simulink library "hdlssclib"  (R2019a)
settings: Solver=VariableStepAuto  StartTime=0.0  StopTime=10.0  RelTol=1e-3
undefined symbols (not defined in the file or in its folder): constMatrix
libraries: $bdroot x4
settings Model: Creator=The MathWorks, Inc.  LastModifiedBy=The MathWorks, Inc.
settings DataIOCC: ReturnWorkspaceOutputs=off
settings DebuggingCC: ArithmeticOperatorsInVariantConditions=warning
settings SFSimCC: SimUseLocalCustomCode=off
settings RTWCC: RTWUseLocalCustomCode=off
settings CodeAppCC: StateflowObjectComments=on
settings GRTTargetCC: TargetLangStandard=C89/C90 (ANSI)
settings ConfigComp: CovMetricSettings=dsw  CovHtmlReporting=on  CovSaveCumulativeToWorkspaceVar=on  CovSaveSingleToWorkspaceVar=on  CovShowResultsExplorer=off  CovExternalEMLEnable=off

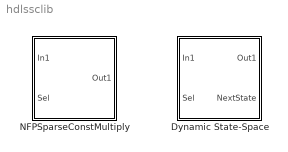
== system hdlssclib ==
  Dynamic State-Space : Subsystem  mask{A=1, B=1, C=1, D=1, X0=0}
      mask prompts: X0 "Initial conditions:"
      mask init:
      | % Dynamic State-Space block configuration
      | % the Dynamic State-Space block has multiple possible configurations based
      | % on the mask parameter values
      | % the Dynamic State-Space block implements the following equations:
      | % NextState     = A * State + B * In1 -> state update equation
      | % Out1          = C * State + D * In1 -> output equation
      | % State <- NextState
      | %
      | % where A, B, C, and D are mask parameters
      | % State represents the current internal state
      | % NextState and Out1 are block outputs
      | % In1 and Sel are block inputs
      | % Sel indexes into dimension 3 of the mask parameters A, B, C, and D
      | 
      | % determine the block configuration from the mask parameter values
      | % three configurations of the Dynamic State-Space block are currently
      | % implemented
      | % configuration 1 - nonzero A,B,C,D
      | % configuration 2 - nonzero A,B,C and zero D
      | % configuration 3 - nonzero D and zero A,B,C
      | 
      | % determine nonzero mask parameters
      | isNonZeroA = any(A(:));
      | isNonZeroB = any(B(:));
      | isNonZeroC = any(C(:));
      | isNonZeroD = any(D(:));
      | 
      | if all([isNonZeroA isNonZeroB isNonZeroC isNonZeroD])
      |     % configuration 1
      |     % x(n+1)    = A*x(n) + B*u(n)
      |     % y(n)      = C*x(n) + D*u(n)
      |     config = 1;
      | elseif all([isNonZeroA isNonZeroB isNonZeroC ~isNonZeroD])
      |     % configuration 2
      |     % x(n+1)    = A*x(n) + B*u(n)
      |     % y(n)      = C*x(n)
      |     config = 2;
      | elseif all([~isNonZeroA ~isNonZeroB ~isNonZeroC isNonZeroD])
      |     % configuration 3
      |     % x(n+1)    = 0
      |     % y(n)      = D*u(n)
      |     config = 3;
      | else
      |     % unimplemented configuration
      |     % default implementation = configuration 1
      |     config = 1;
      | end
      | 
      | % top level block - Dynamic State-Space
      | topBlk = gcb;
      | 
      | % Dynamic State-Space block inports and outports
      | topInports = find_system(topBlk,'LookUnderMasks','all','FollowLinks','on','SearchDepth','1','BlockType','Inport');
      | topOutports = find_system(topBlk,'LookUnderMasks','all','FollowLinks','on','SearchDepth','1','BlockType','Outport');
      | 
      | % blocks inside the Dynamic State-Space block
      | % (not all blocks are present in every configuration)
      | % Name: block name, Position: block position
      | blks = [];
      | % NFPSparseConstMultiply blocks to implement floating point multiplications
      | blks(1).Name = 'NFPMulA';
      | blks(1).Position = [110 170 190 250];
      | blks(2).Name = 'NFPMulB';
      | blks(2).Position = [110 30 190 110];
      | blks(3).Name = 'NFPMulC';
      | blks(3).Position = [410 85 490 165];
      | blks(4).Name = 'NFPMulD';
      | blks(4).Position = [410 -40 490 40];
      | % Sum blocks to implement floating point additions
      | blks(5).Name = 'SumAB';
      | blks(5).Position = [230 55 260 85];
      | blks(6).Name = 'SumCD';
      | blks(6).Position = [520 -15 550 15];
      | % Unit delay block to implement the state
      | blks(7).Name = 'State';
      | blks(7).Position = [295 53 330 87];
      | 
      | % delete all blocks before redrawing
      | nfpMulBlks = find_system(topBlk,'LookUnderMasks','all','FollowLinks','on','SearchDepth','1','ReferenceBlock','hdlssclib/NFPSparseConstMultiply');
      | sumBlks = find_system(topBlk,'LookUnderMasks','all','FollowLinks','on','SearchDepth','1','BlockType','Sum');
      | delayBlks = find_system(topBlk,'LookUnderMasks','all','FollowLinks','on','SearchDepth','1','BlockType','UnitDelay');
      | constBlks = find_system(topBlk,'LookUnderMasks','all','FollowLinks','on','SearchDepth','1','BlockType','Constant');
      | trmtBlks = find_system(topBlk,'LookUnderMasks','all','FollowLinks','on','SearchDepth','1','BlockType','Terminator');
      | deleteBlks = [nfpMulBlks; sumBlks; delayBlks; constBlks; trmtBlks];
      | for ii = 1:numel(deleteBlks)
      |     hLines = get_param(deleteBlks{ii},'LineHandles');
      |     % get connected inport lines. this handles the situation when a block
      |     % inport is unconnected.
      |     inports = hLines.Inport(hLines.Inport ~= -1);
      |     % get connected outport lines. this handles the situation when a block
      |     % outport is unconnected.
      |     outports = hLines.Outport(hLines.Outport ~= -1);
      |     % delete inport connections
      |     delete_line(inports);
      |     % delete outport connections
      |     delete_line(outports);
      |     % delete the block
      |     delete_block(deleteBlks{ii});
      | end
      | 
      | if config == 1
      |     % configuration 1
      |     % x(n+1)    = A*x(n) + B*u(n)
      |     % y(n)      = C*x(n) + D*u(n)
      |     
      |     % add NFPMulA block to perform A*x(n)
      |     add_block('hdlssclib/NFPSparseConstMultiply',[topBlk '/' blks(1).Name],'Position',blks(1).Position);
      |     set_param([topBlk '/' blks(1).Name],'constMatrix','A');
      |     % add NFPMulB block to perform B*u(n)
      |     add_block('hdlssclib/NFPSparseConstMultiply',[topBlk '/' blks(2).Name],'Position',blks(2).Position);
      |     set_param([topBlk '/' blks(2).Name],'constMatrix','B');
      |     % add sum block to perform A*x(n) + B*u(n)
      |     add_block('simulink/Math Operations/Sum',[topBlk '/' blks(5).Name],'Position',blks(5).Position,'InputSameDT','on');
      |     % add unit delay block to store the state
      |     add_block('simulink/Discrete/Unit Delay',[topBlk '/' blks(7).Name],'Position',blks(7).Position);
      |     set_param([topBlk '/' blks(7).Name],'InitialCondition','X0');
      |     % connect NFPMulA and NFPMulB outputs to SumAB inputs
      |     add_line(topBlk,[blks(1).Name '/1'],[blks(5).Name '/2'],'autorouting','on');
      |     add_line(topBlk,[blks(2).Name '/1'],[blks(5).Name '/1'],'autorouting','on');
      |     % connect sumAB output to State input
      |     add_line(topBlk,[blks(5).Name '/1'],[blks(7).Name '/1'],'autorouting','on');
      |     % connect State output to NFPMulA input 'In1'
      |     add_line(topBlk,[blks(7).Name '/1'],[blks(1).Name '/1'],'autorouting','on');
      |     % connect Dynamic State-Space input 'In1' to NFPMulB input 'In1'
      |     add_line(topBlk,[get_param(topInports{1},'Name') '/1'],[blks(2).Name '/1'],'autorouting','on');
      |     % connect Dynamic State-Space input 'Sel' to NFPMulA and NFPMulB inputs
      |     % 'Sel'
      |     add_line(topBlk,[get_param(topInports{2},'Name') '/1'],[blks(1).Name '/2'],'autorouting','on');
      |     add_line(topBlk,[get_param(topInports{2},'Name') '/1'],[blks(2).Name '/2'],'autorouting','on');
      |     % add NFPMulC block to perform C*x(n)
      |     add_block('hdlssclib/NFPSparseConstMultiply',[topBlk '/' blks(3).Name],'Position',blks(3).Position);
      |     set_param([topBlk '/' blks(3).Name],'constMatrix','C');
      |     % add NFPMulD block to perform D*u(n)
      |     add_block('hdlssclib/NFPSparseConstMultiply',[topBlk '/' blks(4).Name],'Position',blks(4).Position);
      |     set_param([topBlk '/' blks(4).Name],'constMatrix','D');
      |     % add sum block to perform C*x(n) + D*u(n)
      |     add_block('simulink/Math Operations/Sum',[topBlk '/' blks(6).Name],'Position',blks(6).Position,'InputSameDT','on');
      |     % connect NFPMulC and NFPMulD outputs to SumCD inputs
      |     add_line(topBlk,[blks(3).Name '/1'],[blks(6).Name '/2'],'autorouting','on');
      |     add_line(topBlk,[blks(4).Name '/1'],[blks(6).Name '/1'],'autorouting','on');
      |     % connect State output to NFPMulC input 'In1'
      |     add_line(topBlk,[blks(7).Name '/1'],[blks(3).Name '/1'],'autorouting','on');
      |     % connect Dynamic State-Space input 'In1' to NFPMulD input 'In1'
      |     add_line(topBlk,[get_param(topInports{1},'Name') '/1'],[blks(4).Name '/1'],'autorouting','on');
      |     % connect Dynamic State-Space input 'Sel' to NFPMulC and NFPMulD inputs
      |     % 'Sel'
      |     add_line(topBlk,[get_param(topInports{2},'Name') '/1'],[blks(3).Name '/2'],'autorouting','on');
      |     add_line(topBlk,[get_param(topInports{2},'Name') '/1'],[blks(4).Name '/2'],'autorouting','on');
      |     % connect State output to Dynamic State-Space output 'NextState'
      |     add_line(topBlk,[blks(7).Name '/1'],[get_param(topOutports{2},'Name') '/1'],'autorouting','on');
      |     % connect SumCD output to Dynamic State-Space output 'Out1'
      |     add_line(topBlk,[blks(6).Name '/1'],[get_param(topOutports{1},'Name') '/1'],'autorouting','on');
      |     
      | elseif config == 2
      |     % configuration 2
      |     % x(n+1)    = A*x(n) + B*u(n)
      |     % y(n)      = C*x(n)
      |     
      |     % add NFPMulA block to perform A*x(n)
      |     add_block('hdlssclib/NFPSparseConstMultiply',[topBlk '/' blks(1).Name],'Position',blks(1).Position);
      |     set_param([topBlk '/' blks(1).Name],'constMatrix','A');
      |     % add NFPMulB block to perform B*u(n)
      |     add_block('hdlssclib/NFPSparseConstMultiply',[topBlk '/' blks(2).Name],'Position',blks(2).Position);
      |     set_param([topBlk '/' blks(2).Name],'constMatrix','B');
      |     % add sum block to perform A*x(n) + B*u(n)
      |     add_block('simulink/Math Operations/Sum',[topBlk '/' blks(5).Name],'Position',blks(5).Position,'InputSameDT','on');
      |     % add unit delay block to store the state
      |     add_block('simulink/Discrete/Unit Delay',[topBlk '/' blks(7).Name],'Position',blks(7).Position);
      |     set_param([topBlk '/' blks(7).Name],'InitialCondition','X0');
      |     % connect NFPMulA and NFPMulB outputs to SumAB inputs
      |     add_line(topBlk,[blks(1).Name '/1'],[blks(5).Name '/2'],'autorouting','on');
      |     add_line(topBlk,[blks(2).Name '/1'],[blks(5).Name '/1'],'autorouting','on');
      |     % connect sumAB output to State input
      |     add_line(topBlk,[blks(5).Name '/1'],[blks(7).Name '/1'],'autorouting','on');
      |     % connect State output to NFPMulA input 'In1'
      |     add_line(topBlk,[blks(7).Name '/1'],[blks(1).Name '/1'],'autorouting','on');
      |     % connect Dynamic State-Space input 'In1' to NFPMulB input 'In1'
      |     add_line(topBlk,[get_param(topInports{1},'Name') '/1'],[blks(2).Name '/1'],'autorouting','on');
      |     % connect Dynamic State-Space input 'Sel' to NFPMulA and NFPMulB inputs
      |     % 'Sel'
      |     add_line(topBlk,[get_param(topInports{2},'Name') '/1'],[blks(1).Name '/2'],'autorouting','on');
      |     add_line(topBlk,[get_param(topInports{2},'Name') '/1'],[blks(2).Name '/2'],'autorouting','on');
      |     % add NFPMulC block to perform C*x(n)
      |     add_block('hdlssclib/NFPSparseConstMultiply',[topBlk '/' blks(3).Name],'Position',blks(3).Position);
      |     set_param([topBlk '/' blks(3).Name],'constMatrix','C');
      |     % connect State output to NFPMulC input 'In1'
      |     add_line(topBlk,[blks(7).Name '/1'],[blks(3).Name '/1'],'autorouting','on');
      |     % connect Dynamic State-Space input 'Sel' to NFPMulC input 'Sel'
      |     add_line(topBlk,[get_param(topInports{2},'Name') '/1'],[blks(3).Name '/2'],'autorouting','on');
      |     % connect State output to Dynamic State-Space output 'NextState'
      |     add_line(topBlk,[blks(7).Name '/1'],[get_param(topOutports{2},'Name') '/1'],'autorouting','on');
      |     % connect NFPMulC output to Dynamic State-Space output 'Out1'
      |     add_line(topBlk,[blks(3).Name '/1'],[get_param(topOutports{1},'Name') '/1'],'autorouting','on');
      |     
      | else
      |     % configuration 3
      |     % x(n+1)    = 0
      |     % y(n)      = D*u(n)
      |     
      |     % add NFPMulD block to perform D*u(n)
      |     add_block('hdlssclib/NFPSparseConstMultiply',[topBlk '/' blks(4).Name],'Position',blks(4).Position);
      |     set_param([topBlk '/' blks(4).Name],'constMatrix','D');
      |     % connect Dynamic State-Space input 'In1' to NFPMulD input 'In1'
      |     add_line(topBlk,[get_param(topInports{1},'Name') '/1'],[blks(4).Name '/1'],'autorouting','on');
      |     % connect Dynamic State-Space input 'Sel' to NFPMulD input 'Sel'
      |     add_line(topBlk,[get_param(topInports{2},'Name') '/1'],[blks(4).Name '/2'],'autorouting','on');
      |     % connect NFPMulD output to Dynamic State-Space output 'Out1'
      |     add_line(topBlk,[blks(4).Name '/1'],[get_param(topOutports{1},'Name') '/1'],'autorouting','on');
      |     % connect Dynamic State-Space output 'NextState' to a constant block
      |     % with 0 value
      |     add_block('simulink/Sources/Constant',[topBlk '/Constant1'],...
      |         'Position',[525 -85 545 -65],...
      |         'Value', '0',...
      |         'SampleTime','-1',...
      |         'OutDataTypeStr','single');
      |     add_line(topBlk,'Constant1/1',[get_param(topOutports{2},'Name') '/1'],'autorouting','on');
      | end
      mask DialogControl StateSpaceParameters Prompt: State-Space Parameters
  NFPSparseConstMultiply : Subsystem  mask{constMatrix=constMatrix}
      mask prompts: constMatrix "Constant matrix:"
      mask init:
      | thisBlk = gcb;
      | 
      | % dimensionality of 'constMatrix'
      | if isempty(constMatrix)
      |     dimsConstMatrix = -1;
      | else
      |     dimsConstMatrix = length(size(constMatrix));
      | end
      | 
      | % find the selector block
      | selectorBlk = [];
      | selectorBlk = find_system(thisBlk, ...
      |     'LookUnderMasks', 'all', ...
      |     'FollowLinks', 'on', ...
      |     'SearchDepth', 1, ...
      |     'Name', 'Selector');
      | 
      | if (dimsConstMatrix == 2)
      |     if ~isempty(selectorBlk)
      |         % delete the selector block
      |         selectorBlkLines = get_param(selectorBlk, 'LineHandles');
      |         delete_line(selectorBlkLines{1}.Inport(1));
      |         delete_line(selectorBlkLines{1}.Inport(2));
      |         delete_line(selectorBlkLines{1}.Outport(1));
      |         delete_block(selectorBlk);
      |         % connect the constant block to the matrix multiply block
      |         add_line(thisBlk, 'Constant/1', 'Product/1', ...
      |             'autorouting', 'on');
      |         % add a terminator block
      |         hTerminatorBlk = add_block('hdlsllib/Sinks/Terminator', ...
      |             strcat(thisBlk, '/Terminator'), ...
      |             'Position', [225 170 255 200]);
      |         % connect the data type conversion block to the terminator block
      |         add_line(thisBlk, 'Data Type Conversion/1', 'Terminator/1', ...
      |             'autorouting', 'on');
      |     end
      | elseif (dimsConstMatrix == 3)
      |     if isempty(selectorBlk)
      |         % delete the terminator block
      |         terminatorBlkLines = get_param(strcat(thisBlk, '/Terminator'), 'LineHandles');
      |         delete_line(terminatorBlkLines.Inport(1));
      |         delete_block(strcat(thisBlk, '/Terminator'));
      |         % disconnect the constant block and matrix multiply block
      |         constantBlkLines = get_param(strcat(thisBlk, '/Constant'), 'LineHandles');
      |         delete_line(constantBlkLines.Outport(1));
      |         % add the selector block
      |         hSelectorBlk = add_block('hdlsllib/Signal Routing/Selector', ...
      |             strcat(thisBlk, '/Selector'), ...
      |             'Position', [260 116 300 154], ...
      |             'NumberOfDimensions', '3', ...
      |             'IndexMode', 'Zero-based', ...
      |             'IndexOptionArray', [{'Select all'}; {'Select all'}; {'Starting index (port)'}], ...
      |             'OutputSizeArray', [{'1'} {'1'} {'1'}]);
      |         % connect the constant block to the selector block
      |         add_line(thisBlk, 'Constant/1', 'Selector/1', ...
      |             'autorouting', 'on');
      |         % connect the data type conversion block to the selector block
      |         add_line(thisBlk, 'Data Type Conversion/1', 'Selector/2', ...
      |             'autorouting', 'on');
      |         % connect the selector block to the matrix multiply block
      |         add_line(thisBlk, 'Selector/1', 'Product/1', ...
      |             'autorouting', 'on');
      |     end
      | else
      |     error(['''Constant matrix'' parameter must be a 2-dimensional or 3-dimensional matrix.']);
      | end

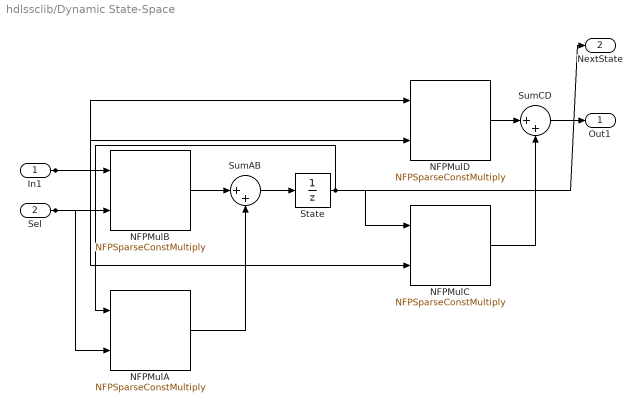
== system hdlssclib/Dynamic State-Space ==
  In1 : Inport
  Sel : Inport  Port=2
  NFPMulA : $bdroot/NFPSparseConstMultiply  constMatrix=A
  NFPMulB : $bdroot/NFPSparseConstMultiply  constMatrix=B
  NFPMulC : $bdroot/NFPSparseConstMultiply  constMatrix=C
  NFPMulD : $bdroot/NFPSparseConstMultiply  constMatrix=D
  State : UnitDelay  InitialCondition=X0  SampleTime=-1  HasFrameUpgradeWarning=on
  SumAB : Sum  Inputs=|++  InputSameDT=on
  SumCD : Sum  Inputs=|++  InputSameDT=on
  Out1 : Outport
  NextState : Outport  Port=2
  wires:
  NFPMulA/1 -> SumAB/2
  NFPMulB/1 -> SumAB/1
  SumAB/1 -> State/1
  State/1 -> NFPMulA/1, NFPMulC/1, NextState/1
  In1/1 -> NFPMulB/1, NFPMulD/1
  Sel/1 -> NFPMulA/2, NFPMulB/2, NFPMulC/2, NFPMulD/2
  NFPMulC/1 -> SumCD/2
  NFPMulD/1 -> SumCD/1
  SumCD/1 -> Out1/1

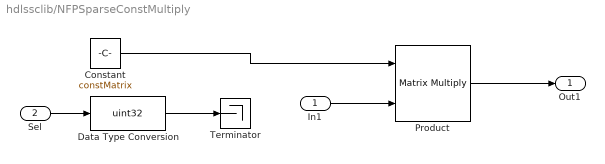
== system hdlssclib/NFPSparseConstMultiply ==
  In1 : Inport  PortDimensions=[size(constMatrix, 2), 1]
  Sel : Inport  Port=2  PortDimensions=1
  Constant : Constant  Value=constMatrix  VectorParams1D=off  OutDataTypeStr=Inherit: Inherit via back propagation  SampleTime=-1
  Data Type Conversion : DataTypeConversion  OutDataTypeStr=uint32  RndMeth=Nearest
  Product : Product  Multiplication=Matrix(*)  InputSameDT=on
  Terminator : Terminator
  Out1 : Outport
  wires:
  In1/1 -> Product/2
  Product/1 -> Out1/1
  Sel/1 -> Data Type Conversion/1
  Constant/1 -> Product/1
  Data Type Conversion/1 -> Terminator/1
